simulink model "BevDriveCycleModel"  (R2020b)
settings: Solver=ode23t  StartTime=0.0  StopTime=2474  MaxStep=0.1  RelTol=1e-3  AbsTol=1e-3  EnableMultiTasking=on
PreLoadFcn:
  | BevDriveCycleBasic_params
libraries: fl_lib x1, nesl_utility x1
Description:
  | Battery Electric Vehicle drive cycle simulation
settings Model: FPTRunName=Active  Creator=MathWorks  LastModifiedBy=isaacito
settings SolverCC: AutoScaleAbsTol=off  MinimalZcImpactIntegration=on
settings DataIOCC: MaxDataPoints=15000  SaveFormat=Array
settings OptimizationCC: ExpressionDepthLimit=2147483647  LifeSpan=inf
settings DebuggingCC: UnderspecifiedInitializationDetection=Classic  MergeDetectMultiDrivingBlocksExec=none  FcnCallInpInsideContextMsg=warning  StateNameClashWarn=warning  SFUnexpectedBacktrackingDiag=warning  SFNoUnconditionalDefaultTransitionDiag=warning  SFExecutionAtInitializationDiag=none  ArithmeticOperatorsInVariantConditions=warning
settings HardwareCC: ProdBitPerPointer=32  ProdBitPerSizeT=32  ProdBitPerPtrDiffT=32  ProdLargestAtomicFloat=None  ProdIntDivRoundTo=Undefined  ProdEndianess=Unspecified  ProdWordSize=32  ProdHWDeviceType=32-bit Generic
settings ModelReferenceCC: PropagateSignalLabelsOutOfModel=off
settings SFSimCC: SimUseLocalCustomCode=off  CustomCodeUndefinedFunction=UseInterfaceOnly
settings RTWCC: RTWUseLocalCustomCode=off
settings CodeAppCC: StateflowObjectComments=on
settings GRTTargetCC: TargetLangStandard=C89/C90 (ANSI)  CombineOutputUpdateFcns=off  GRTInterface=on
settings ConfigComp: CovScope=Subsystem  CovPath=Driver & Environment/Torque Limiter  CovMetricSettings=dcmw  CovSaveCumulativeToWorkspaceVar=on  CovSaveSingleToWorkspaceVar=on  CovExternalEMLEnable=off
settings SimscapeCC: SimscapeNominalValues="[{\"value\":\"20\",\"unit\":\"A\"},{\"value\":\"1\",\"unit\":\"bar\"},{\"value\":\"1\",\"unit\":\"cm^2\"},{\"value\":\"1\",\"unit\":\"cm^3/s\"},{\"value\":\"1\",\"unit\":\"kJ/kg\"},{\"value\":\"1\",\"unit\":\"kW\"},{\"value\":\"1\",\"unit\":\"l\"},{\"value\":\"1\",\"unit\":\"N\"},{\"value\":\"40\",\"unit\":\"N*m\"},{\"value\":\"350\",\"unit\":\"V\"}]"  SimscapeLogType=all  SimscapeLogSimulationStatistics=on  SimscapeLogName=logoutssc  SimscapeLogLimitData=off  SimscapeLogDataHistory=10000

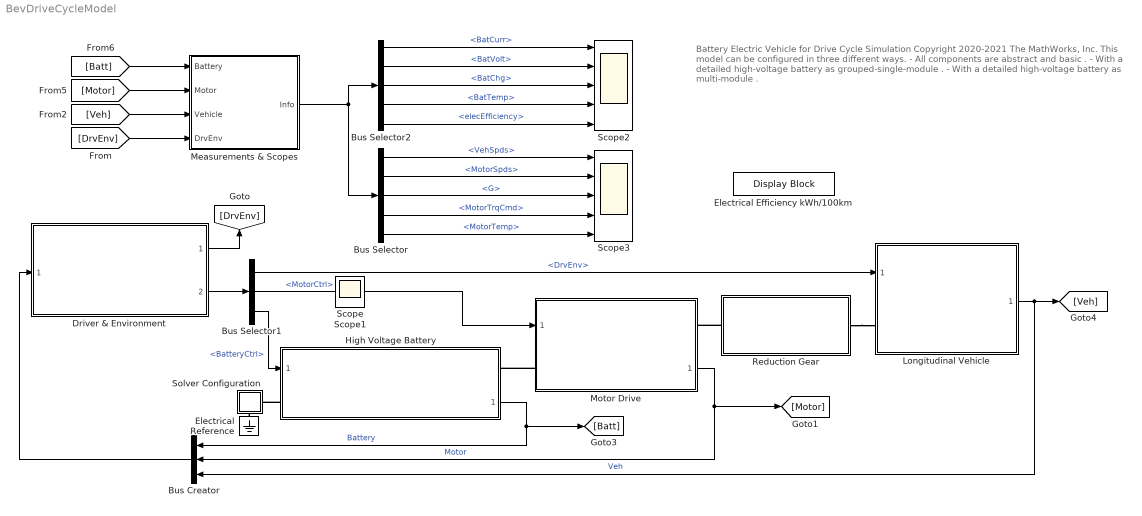
== system BevDriveCycleModel ==
  note: Battery Electric Vehicle for Drive Cycle Simulation
      |
      | Copyright 2020-2021 The MathWorks, Inc.
      |
      | This model can be configured in three different ways.
      | - All components are abstract and basic .
      | - With a detailed high-voltage battery as grouped-single-module .
      | - With a detailed high-voltage battery as multi-module .
  Bus Creator : BusCreator  Inputs=3
  Bus Selector : BusSelector  OutputSignals=VehSpds,MotorSpds,G,MotorTrqCmd,MotorTemp
  Bus Selector1 : BusSelector  OutputSignals=DrvEnv,MotorCtrl,BatteryCtrl
  Bus Selector2 : BusSelector  OutputSignals=BatCurr,BatVolt,BatChg,BatTemp,elecEfficiency
  Driver & Environment : Subsystem  ReferencedSubsystem=DirectDriveCycleBasicRefSub
  Electrical Reference : fl_lib/Electrical/Electrical Elements/Electrical Reference
  Electrical Efficiency kWh/100km : DisplayBlock  LabelPosition=Bottom  Format=Custom  Transparency=1  Opacity=0.5  FormatString=%4.1f
  High Voltage Battery : Subsystem  ReferencedSubsystem=BatteryHighVoltageBasic_refsub
      settings: PortSchema="{\"entries\":[{\"content\":{\"sides\":[{\"content\":{\"connectorIds\":[\"In1\",\"LConn1\"]},\"type\":\"ConnectorPlacement.EquallySpacedRectSide\",\"uuid\":\"5db791d4-e733-413a-9b9b-d79e76ac9bb0\"},{\"content\":{\"connectorIds\":[\"RConn1\",\"Out1\"],\"side\":\"RIGHT\"},\"type\":\"ConnectorPlacement.EquallySpacedRectSide\",\"uuid\":\"0c12beb5-1dc0-4de1-849a-92aaa1061486\"},{\"content\":{\"connectorIds\":[],\"side\":\"TOP\"},\"type\":\"ConnectorPlacement.EquallySpacedRectSide\",\"uuid\":\"758dbf8c-c8ee-4b73-af05-227531b6198b\"},{\"content\":{\"connectorIds\":[],\"side\":\"HIDDEN\"},\"type\":\"ConnectorPlacement.EquallySpacedRectSide\",\"uuid\":\"fa4920b8-ec2a-4218-a476-41d1e0d36381\"}]},\"type\":\"ConnectorPlacement.EquallySpacedConnector\",\"uuid\":\"d828a3e3-8826-44df-b770-75b0ad7bf91b\"}],\"packageUris\":[\"http://schema.mathworks.com/mf0/Connector/R2020b\"],\"version\":\"1.0\"}"
  Longitudinal Vehicle : Subsystem  ReferencedSubsystem=Vehicle1DBasicRefSub
  Measurements & Scopes : Subsystem
  Motor Drive : Subsystem  ReferencedSubsystem=MotorDriveBasicRefSub
      settings: PortSchema="{\"entries\":[{\"content\":{\"sides\":[{\"content\":{\"connectorIds\":[\"In1\",\"LConn1\"]},\"type\":\"ConnectorPlacement.EquallySpacedRectSide\",\"uuid\":\"c1f5a59b-528f-494b-9e01-fc912b1a17eb\"},{\"content\":{\"connectorIds\":[\"RConn1\",\"Out1\"],\"side\":\"RIGHT\"},\"type\":\"ConnectorPlacement.EquallySpacedRectSide\",\"uuid\":\"75d4d618-93a2-4221-89a4-eaa0aa688ad9\"},{\"content\":{\"connectorIds\":[],\"side\":\"TOP\"},\"type\":\"ConnectorPlacement.EquallySpacedRectSide\",\"uuid\":\"16e45e4e-5af9-4938-aa9b-3d67492021aa\"},{\"content\":{\"connectorIds\":[],\"side\":\"HIDDEN\"},\"type\":\"ConnectorPlacement.EquallySpacedRectSide\",\"uuid\":\"b3ebe272-24a1-414f-bf44-13c1d02686eb\"}]},\"type\":\"ConnectorPlacement.EquallySpacedConnector\",\"uuid\":\"4cf231c1-c51e-4d56-b7c0-db761ab55f01\"}],\"packageUris\":[\"http://schema.mathworks.com/mf0/Connector/R2020b\"],\"version\":\"1.0\"}"
  Reduction Gear : Subsystem  ReferencedSubsystem=ReducerBasicRefSub
  Scope2 : Scope  NumInputPorts=5
  Scope3 : Scope  NumInputPorts=5
  Solver Configuration : Subsystem
      settings: PortSchema="{\"entries\":[{\"content\":{\"sides\":[{\"content\":{\"connectorIds\":[]},\"type\":\"ConnectorPlacement.EquallySpacedRectSide\",\"uuid\":\"4a7e26c2-e9e9-4fea-b605-533b1a682be7\"},{\"content\":{\"connectorIds\":[\"RConn1\"],\"side\":\"RIGHT\"},\"type\":\"ConnectorPlacement.EquallySpacedRectSide\",\"uuid\":\"0210e324-555e-4372-b836-fcc8ab23e933\"},{\"content\":{\"connectorIds\":[],\"side\":\"TOP\"},\"type\":\"ConnectorPlacement.EquallySpacedRectSide\",\"uuid\":\"9bbae011-e6fc-4534-a44f-d79a5697c939\"},{\"content\":{\"connectorIds\":[\"RConn2\"],\"side\":\"BOTTOM\"},\"type\":\"ConnectorPlacement.EquallySpacedRectSide\",\"uuid\":\"d5829c0a-26ea-402d-a1c6-900997ddf1a8\"}]},\"type\":\"ConnectorPlacement.EquallySpacedConnector\",\"uuid\":\"f4e17c65-54c6-42fe-a467-9c6b014b697a\"}],\"packageUris\":[\"http://schema.mathworks.com/mf0/Connector/19700101\"],\"version\":\"1.0\"}"
  Scope : Scope
  Scope1 : Scope
  wires:
  [Veh] -> Measurements & Scopes/3(Vehicle)
  [Motor] -> Measurements & Scopes/2(Motor)
  [Batt] -> Measurements & Scopes/1(Battery)
  High Voltage Battery/1 -> [Batt], Bus Creator/1  "Battery"
  Longitudinal Vehicle/1 -> [Veh], Bus Creator/3  "Veh"
  [DrvEnv] -> Measurements & Scopes/4(DrvEnv)
  Driver & Environment/1 -> [DrvEnv]
  Bus Selector1/2 -> Motor Drive/1  "<MotorCtrl>"
  Bus Selector/1 -> Scope3/1  "<VehSpds>"
  Bus Selector/2 -> Scope3/2  "<MotorSpds>"
  Bus Selector/3 -> Scope3/3  "<G>"
  Bus Selector/4 -> Scope3/4  "<MotorTrqCmd>"
  Motor Drive/1 -> [Motor], Bus Creator/2  "Motor"
  Bus Creator/1 -> Driver & Environment/1
  Bus Selector1/3 -> High Voltage Battery/1  "<BatteryCtrl>"
  Driver & Environment/2 -> Bus Selector1/1
  Bus Selector1/1 -> Longitudinal Vehicle/1  "<DrvEnv>"
  Bus Selector/5 -> Scope3/5  "<MotorTemp>"
  Bus Selector2/2 -> Scope2/2  "<BatVolt>"
  Bus Selector2/4 -> Scope2/4  "<BatTemp>"
  Bus Selector2/5 -> Scope2/5  "<elecEfficiency>"
  Bus Selector2/3 -> Scope2/3  "<BatChg>"
  Bus Selector2/1 -> Scope2/1  "<BatCurr>"
  Measurements & Scopes/1(Info) -> Bus Selector/1, Bus Selector2/1
  connections:
  Reduction Gear/LConn1 -- Motor Drive/RConn1
  Reduction Gear/RConn1 -- Longitudinal Vehicle/LConn1
  Motor Drive/LConn1 -- High Voltage Battery/RConn1
  High Voltage Battery/LConn1 -- Solver Configuration/RConn1
  Electrical Reference/LConn1 -- Solver Configuration/RConn2

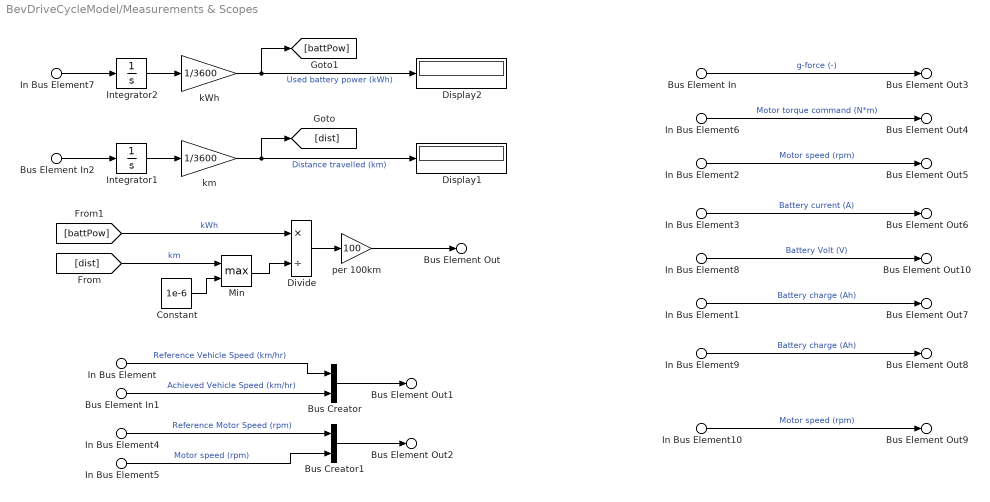
== system BevDriveCycleModel/Measurements & Scopes ==
  In Bus Element3 : Inport  PortName=Battery  Element=Current
  In Bus Element1 : Inport  PortName=Battery  Element=Charge
  In Bus Element7 : Inport  PortName=Battery  Element=Power
      settings: AttributesFormatString=%<Unit>
  In Bus Element9 : Inport  PortName=Battery  Element=BatTemp
  In Bus Element8 : Inport  PortName=Battery  Element=Volt
  In Bus Element6 : Inport  Port=2  PortName=Motor  Element=TrqCmd
      settings: AttributesFormatString=%<Unit>
  In Bus Element5 : Inport  Port=2  PortName=Motor  Element=MotorSpd
      settings: AttributesFormatString=%<Unit>
  In Bus Element2 : Inport  Port=2  PortName=Motor  Element=MotorSpd
      settings: AttributesFormatString=%<Unit>
  In Bus Element10 : Inport  Port=2  PortName=Motor  Element=Temp
      settings: AttributesFormatString=%<Unit>
  Bus Element In : Inport  Port=3  PortName=Vehicle  Element=G
  Bus Element In2 : Inport  Port=3  PortName=Vehicle  Element=VehSpd
      settings: AttributesFormatString=%<Unit>
  Bus Element In1 : Inport  Port=3  PortName=Vehicle  Element=VehSpd
      settings: AttributesFormatString=%<Unit>
  In Bus Element : Inport  Port=4  PortName=DrvEnv  Element=VehSpdRef
  In Bus Element4 : Inport  Port=4  PortName=DrvEnv  Element=MotorSpdRef
  Bus Creator : BusCreator  Inputs=2
  Bus Creator1 : BusCreator  Inputs=2
  Constant : Constant  Value=1e-6
  Display1 : Display
  Display2 : Display
  Divide : Product  Inputs=*/
  Integrator1 : Integrator
  Integrator2 : Integrator
  Min : MinMax  Function=max  Inputs=2
  kWh : Gain  Gain=1/3600
  km : Gain  Gain=1/3600
  per 100km : Gain  Gain=100
  Bus Element Out : Outport  PortName=Info  Element=elecEfficiency
      settings: AttributesFormatString=%<Unit>
  Bus Element Out1 : Outport  PortName=Info  Element=VehSpds
      settings: AttributesFormatString=%<Unit>
  Bus Element Out2 : Outport  PortName=Info  Element=MotorSpds
      settings: AttributesFormatString=%<Unit>
  Bus Element Out3 : Outport  PortName=Info  Element=G
      settings: AttributesFormatString=%<Unit>
  Bus Element Out4 : Outport  PortName=Info  Element=MotorTrqCmd
      settings: AttributesFormatString=%<Unit>
  Bus Element Out5 : Outport  PortName=Info  Element=MotorSpd
      settings: AttributesFormatString=%<Unit>
  Bus Element Out6 : Outport  PortName=Info  Element=BatCurr
      settings: AttributesFormatString=%<Unit>
  Bus Element Out7 : Outport  PortName=Info  Element=BatChg
      settings: AttributesFormatString=%<Unit>
  Bus Element Out8 : Outport  PortName=Info  Element=BatTemp
      settings: AttributesFormatString=%<Unit>
  Bus Element Out9 : Outport  PortName=Info  Element=MotorTemp
      settings: AttributesFormatString=%<Unit>
  Bus Element Out10 : Outport  PortName=Info  Element=BatVolt
      settings: AttributesFormatString=%<Unit>
  wires:
  In Bus Element1/1 -> Bus Element Out7/1  "Battery charge (Ah)"
  In Bus Element3/1 -> Bus Element Out6/1  "Battery current (A)"
  Bus Element In2/1 -> Integrator1/1
  Integrator1/1 -> km/1
  km/1 -> [dist], Display1/1  "Distance travelled (km)"
  In Bus Element7/1 -> Integrator2/1
  Integrator2/1 -> kWh/1
  kWh/1 -> [battPow], Display2/1  "Used battery power (kWh)"
  [battPow] -> Divide/1  "kWh"
  Divide/1 -> per 100km/1
  In Bus Element/1 -> Bus Creator/1  "Reference Vehicle Speed (km/hr)"
  Bus Element In1/1 -> Bus Creator/2  "Achieved Vehicle Speed (km/hr)"
  In Bus Element5/1 -> Bus Creator1/2  "Motor speed (rpm)"
  In Bus Element4/1 -> Bus Creator1/1  "Reference Motor Speed (rpm)"
  [dist] -> Min/1  "km"
  Min/1 -> Divide/2
  Constant/1 -> Min/2
  Bus Creator1/1 -> Bus Element Out2/1
  In Bus Element2/1 -> Bus Element Out5/1  "Motor speed (rpm)"
  per 100km/1 -> Bus Element Out/1
  Bus Element In/1 -> Bus Element Out3/1  "g-force (-)"
  Bus Creator/1 -> Bus Element Out1/1
  In Bus Element6/1 -> Bus Element Out4/1  "Motor torque command (N*m)"
  In Bus Element9/1 -> Bus Element Out8/1  "Battery charge (Ah)"
  In Bus Element10/1 -> Bus Element Out9/1  "Motor speed (rpm)"
  In Bus Element8/1 -> Bus Element Out10/1  "Battery Volt (V)"

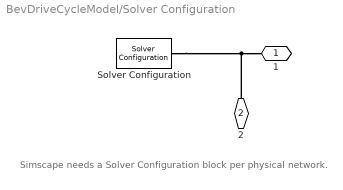
== system BevDriveCycleModel/Solver Configuration ==
  note: Simscape needs a Solver Configuration block per physical network.
  Solver Configuration : nesl_utility/Solver Configuration  PhysicalDomain=network_engine_domain  SubClassName=solver  LeftPortType=input  RightPortType=generic  Tones=[]  Harmonics=[]  SimulateNoise=off  Profile=off  UseLocalSampling=off  EnableSwitchedLinearOptims=on  FrequencyDomain=off  UseCCode=off  RelTol=0.001  AbsTol=1e-06  MinStep=1e-09  ToWorkspace=off  RevertToSquareIcSolve=off  NumHomotopyIterations=100  PhasorMode=off  PhasorModeNumHarmonics=1  DoDC=off  ResidualTolerance=1e-6  UseLocalSolver=off  LocalSolverChoice=NE_BACKWARD_EULER_ADVANCER  LocalSolverSampleTime=0.01  DoFixedCost=off  MaxNonlinIter=3  MaxModeIter=2  ComputeImpulses=off  ImpulseIterations=2  LinearAlgebra=auto  EquationFormulation=NE_TIME_EF  DelaysMemoryBudget=1024  AutomaticFiltering=on  FilteringTimeConstant=0.001  PartitionStorageMethod=AS_NEEDED  PartitionMemoryBudget=1024  PartitionMethod=FAST
      settings: AttributesFormatString=Local solver %<UseLocalSolver>
  1 : PMIOPort  Side=Right
  2 : PMIOPort  Port=2  Side=Right
  connections:
  Solver Configuration/RConn1 -- 1/RConn1 -- 2/RConn1
